simulink model "Paddles"  (R2025b)
settings: configuration reference "VehicleFixed1ms" (kept outside this file)
libraries: autolibutils x2, simulink x1
settings Model: DataDictionary=VirtualMotoTemplate.sldd  ModifiedByFormat=The MathWorks, Inc.  Creator=The MathWorks, Inc.  LastModifiedBy=The MathWorks, Inc.
settings ConfigSetRef: SourceName=VehicleFixed1ms

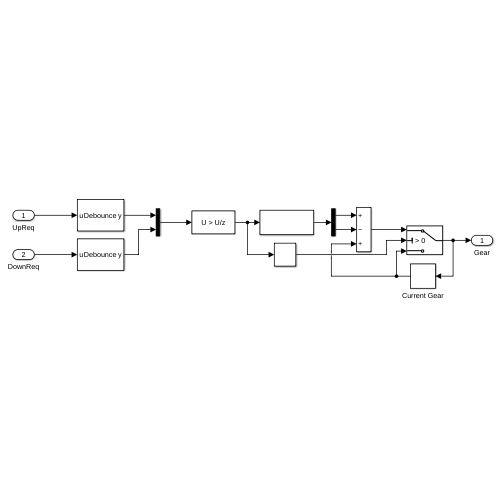
[thumbnail: Simulink's stored preview of the top-level diagram]
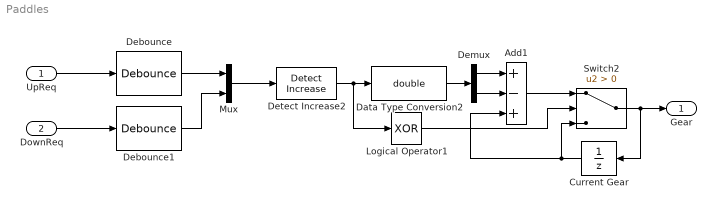
== system Paddles ==
  UpReq : Inport
  DownReq : Inport  Port=2  Unit=rad/s
  Add1 : Sum  Inputs=+-+
  Current Gear : UnitDelay  SampleTime=-1  HasFrameUpgradeWarning=on
  Data Type Conversion2 : DataTypeConversion  OutDataTypeStr=double  SaturateOnIntegerOverflow=off  RndMeth=Floor
  Debounce : autolibutils/Debounce  DbcOn_Cnts=10  DbcOff_Cnts=10  aMode=aMode
  Debounce1 : autolibutils/Debounce  DbcOn_Cnts=10  DbcOff_Cnts=10  aMode=aMode
  Demux : Demux  Outputs=2
  Detect Increase2 : simulink/Logic and Bit Operations/Detect Increase  vinit=0.0  OutDataTypeStr=boolean
  Logical Operator1 : Logic  Operator=XOR  Inputs=1  AllPortsSameDT=off  OutDataTypeStr=boolean
  Mux : Mux  Inputs=2
  Switch2 : Switch  Criteria=u2 > Threshold  SaturateOnIntegerOverflow=off  InputSameDT=off
  Gear : Outport  VectorParamsAs1DForOutWhenUnconnected=off
  wires:
  Demux/2 -> Add1/2
  Debounce/1 -> Mux/1
  Debounce1/1 -> Mux/2
  UpReq/1 -> Debounce/1
  Detect Increase2/1 -> Logical Operator1/1, Data Type Conversion2/1
  Mux/1 -> Detect Increase2/1
  Add1/1 -> Switch2/1
  DownReq/1 -> Debounce1/1
  Data Type Conversion2/1 -> Demux/1
  Switch2/1 -> Current Gear/1, Gear/1
  Logical Operator1/1 -> Switch2/2
  Current Gear/1 -> Switch2/3, Add1/3
  Demux/1 -> Add1/1
